simulink model "Conv_16_12"  (R2016b)
settings: Solver=FixedStepDiscrete  StartTime=0.0  StopTime=10.0  RelTol=1e-3
libraries: hdlsllib x1
settings Model: DataTypeOverride=Off  Creator=ppradhan  LastModifiedBy=ppradhan
settings DataIOCC: SaveOutput=off  SaveTime=off
settings OptimizationCC: BlockReduction=off  ConditionallyExecuteInputs=off  DefaultParameterBehavior=Inlined
settings DebuggingCC: AlgebraicLoopMsg=error  SingleTaskRateTransMsg=error  StrictBusMsg=ErrorOnBusTreatedAsVector
settings HardwareCC: ProdBitPerPointer=32  ProdBitPerSizeT=32  ProdBitPerPtrDiffT=32  ProdLargestAtomicFloat=None  ProdIntDivRoundTo=Undefined  ProdEndianess=Unspecified  ProdWordSize=32  ProdHWDeviceType=ASIC/FPGA->ASIC/FPGA  ProdEqTarget=off

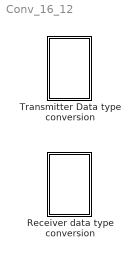
== system Conv_16_12 ==
  Receiver data type conversion : Subsystem
  Transmitter Data type conversion : Subsystem

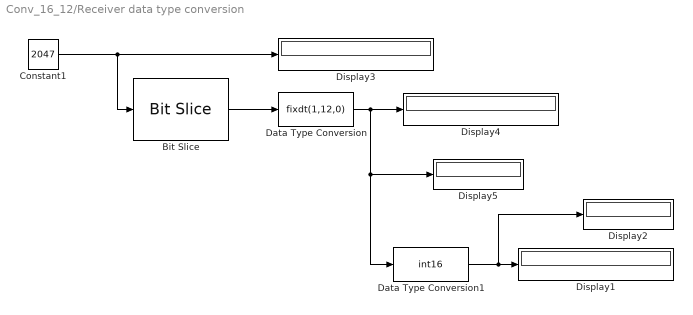
== system Conv_16_12/Receiver data type conversion ==
  Bit Slice : hdlsllib/HDL Operations/Bit Slice  lidx=11  ridx=0
  Constant1 : Constant  Value=2047  OutDataTypeStr=int16  SampleTime=-1
  Data Type Conversion : DataTypeConversion  OutDataTypeStr=fixdt(1,12,0)
  Data Type Conversion1 : DataTypeConversion  OutDataTypeStr=int16
  Display{1..5} (5 alike) : Display
      Display1 settings: Format=binary (Stored Integer)
      Display3 settings: Format=binary (Stored Integer)
      Display4 settings: Format=binary (Stored Integer)
  wires:
  Bit Slice/1 -> Data Type Conversion/1
  Data Type Conversion1/1 -> Display2/1, Display1/1
  Data Type Conversion/1 -> Data Type Conversion1/1, Display5/1, Display4/1
  Constant1/1 -> Bit Slice/1, Display3/1

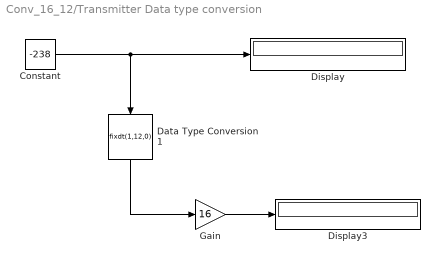
== system Conv_16_12/Transmitter Data type conversion ==
  Constant : Constant  Value=-238  OutDataTypeStr=fixdt(1,12)  SampleTime=-1
  Data Type Conversion1 : DataTypeConversion  OutDataTypeStr=fixdt(1,12,0)  ConvertRealWorld=Stored Integer (SI)
  Display : Display
      settings: Format=binary (Stored Integer)
  Display3 : Display
      settings: Format=binary (Stored Integer)
  Gain : Gain  Gain=16  ParamDataTypeStr=fixdt(0,5,0)  OutDataTypeStr=fixdt(1,16,0)
  wires:
  Constant/1 -> Display/1, Data Type Conversion1/1
  Gain/1 -> Display3/1
  Data Type Conversion1/1 -> Gain/1
